simulink library "Compressor_Alpha"  (R2019b)
settings: Solver=ode45  StartTime=0.0  StopTime=10.0  RelTol=1e-3  EnableMultiTasking=on
undefined symbols (not defined in the file): Comp
libraries: $bdroot x4, simulink x1
settings Model: Creator=mbrauer  LastModifiedBy=bhisma
settings DataIOCC: LimitDataPoints=on  SaveFormat=Array  SignalLoggingSaveFormat=ModelDataLogs  ReturnWorkspaceOutputs=off
settings OptimizationCC: LifeSpan=inf
settings DebuggingCC: SolverPrmCheckMsg=warning  MultiTaskDSMMsg=warning  MultiTaskCondExecSysMsg=none  SFUnexpectedBacktrackingDiag=warning  SFNoUnconditionalDefaultTransitionDiag=warning  SFExecutionAtInitializationDiag=none  ArithmeticOperatorsInVariantConditions=warning
settings HardwareCC: ProdBitPerPointer=32  ProdBitPerSizeT=32  ProdBitPerPtrDiffT=32  ProdLargestAtomicFloat=None  ProdIntDivRoundTo=Undefined  ProdEndianess=Unspecified  ProdWordSize=32  ProdHWDeviceType=32-bit Generic
settings ModelReferenceCC: PropagateSignalLabelsOutOfModel=off
settings SFSimCC: SimUseLocalCustomCode=off  CustomCodeUndefinedFunction=UseInterfaceOnly
settings RTWCC: RTWUseLocalCustomCode=off
settings CodeAppCC: StateflowObjectComments=on
settings GRTTargetCC: TargetLangStandard=C89/C90 (ANSI)  GeneratePreprocessorConditionals=Disable all
settings ConfigComp: CovMetricSettings=dw  CovHtmlReporting=on  CovSaveCumulativeToWorkspaceVar=on  CovSaveSingleToWorkspaceVar=on  CovExternalEMLEnable=off

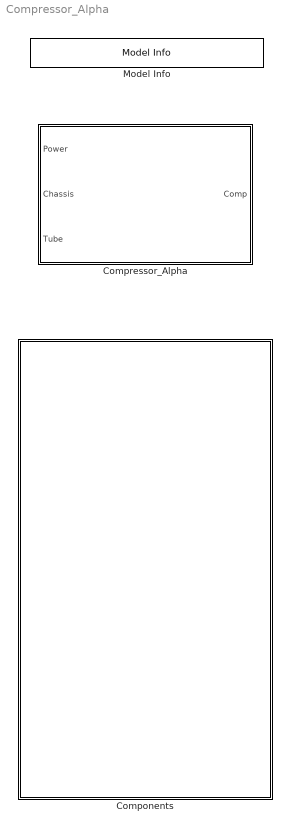
== system Compressor_Alpha ==
  Components : Subsystem
  Compressor_Alpha : Subsystem
  Model Info : simulink/Model-Wide Utilities/Model Info  Frame=on  DisplayStringWithTags=Copyright 2013-2014 The MathWorks, Inc.  HorizontalTextAlignment=Center  LeftAlignmentValue=0.5

== system Compressor_Alpha/Components ==
  Compressor : Subsystem  mask(Compressor){CPR=21, nc=0.75}
      mask prompts: CPR "Compression Ratio"; nc "Efficiency"
      mask help:
      | Basic compressor model, including electric motor.
      |
      | Determines output air pressure and temperature based on defined Compression ratio. Also determines required electrical power.
      mask init:
      | if or(nc > 1,nc<=0)
      |     error('nc should be a value between 0 and 1')
      | end
      | 
      | cp_air = 1e3; 
      | gamma = 1.4;
      mask Display: image('CompressorIcon.png',[80 30 110 140])
  Intercooler : Subsystem  mask(Intercooler){T_air_out=300, eff=0.6}
      mask prompts: T_air_out "Target Output Temperature"; eff "Efficiency"
      mask help:
      | Basic intercooler model, for air to water heat exchange
      |
      | Calculates power to cool input air to desired temperature and converts that heat to water/steam.
      mask init:
      | cp_air      = 1e3;     % kJ/kg/K
      | cp_gas      = 1.996e3; % steam kJ/kg/K
      | cp_liquid   = 4.186e3; % water kJ/kg/K
      | cp_L2G      = 40.7e6/18; % kJ/kg (40.7 kJ/mol / 18 g/mol)
      | T_0         = 273;
      | T_c         = 373;
      | T_max       = 800;
      | maxEnth_liquid = (T_c-T_0)*cp_liquid;
      | minEnth_gas    = maxEnth_liquid+cp_L2G;
      | maxEnth_gas    = minEnth_gas+(T_max-T_c)*cp_gas;
      | if or(eff > 1,eff<=0)
      |     error('eff should be a value between 0 and 1')
      | end
      mask Display: image('Intercooler.png',[60 10 170 180])

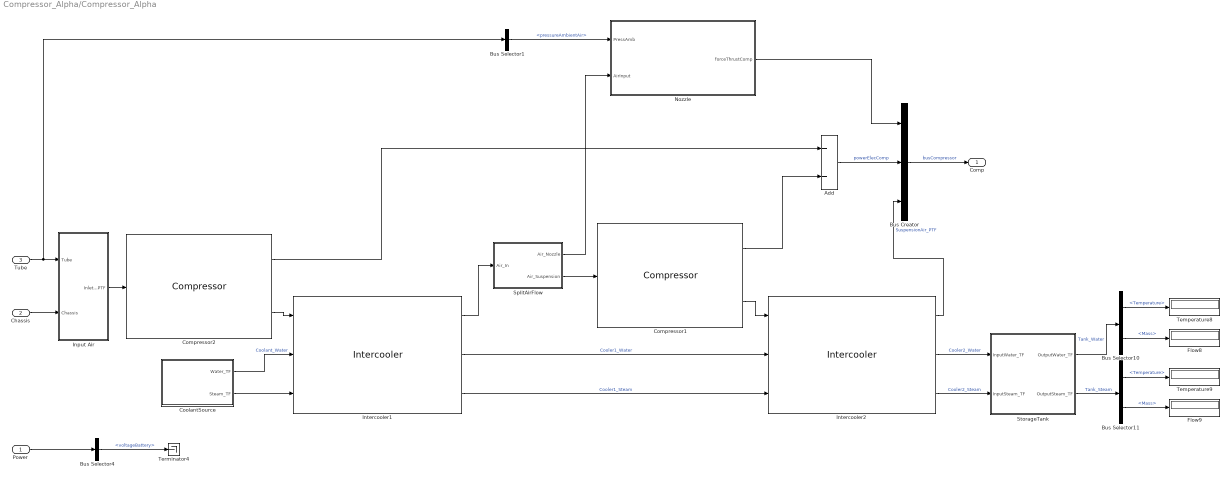
== system Compressor_Alpha/Compressor_Alpha ==
  Power : Inport
  Chassis : Inport  Port=2
  Tube : Inport  Port=3
  Add : Sum  Inputs=--
  Bus Creator : BusCreator  Inputs=3  NonVirtualBus=on
  Bus Selector1 : BusSelector  OutputSignals=pressureAmbientAir
  Bus Selector10 : BusSelector  OutputSignals=Temperature,Mass
  Bus Selector11 : BusSelector  OutputSignals=Temperature,Mass
  Bus Selector4 : BusSelector  OutputSignals=voltageBattery
  Compressor1 : $bdroot/Components/Compressor  CPR=21  nc=0.75
  Compressor2 : $bdroot/Components/Compressor  CPR=21  nc=0.75
  CoolantSource : Subsystem
  Flow8 : Display
      settings: Decimation=100
  Flow9 : Display
      settings: Decimation=100
  Input Air : Subsystem
  Intercooler1 : $bdroot/Components/Intercooler  T_air_out=300  eff=0.6
  Intercooler2 : $bdroot/Components/Intercooler  T_air_out=300  eff=0.6
  Nozzle : Subsystem
  SplitAirFlow : Subsystem
  StorageTank : Subsystem  mask(Liquid/Gas Storage Tank){}
      mask help:
      | This block takes in Flow of a liquid and gas at input temperatures.
      |
      | It accumulates the enthalphy and mass provided and determines a
      | final combination of liquid and gas at proper temperatures.
      |
      | Output should generally be (1) all liquid (2) all gas or (3) a
      | combination of liquid and gas at the boiling point.
      mask init:
      | cp_gas      = 1.996e3; % steam kJ/kg/K
      | cp_liquid   = 4.186e3; % water kJ/kg/K
      | cp_L2G      = 40.7e6/18; % kJ/kg (40.7 kJ/mol / 18 g/mol)
      | T_0         = 273;
      | T_c         = 373;
      | T_max       = 800;
      | maxEnth_liquid = (T_c-T_0)*cp_liquid;
      | minEnth_gas    = maxEnth_liquid+cp_L2G;
      | maxEnth_gas    = minEnth_gas+(T_max-T_c)*cp_gas;
  Temperature8 : Display
      settings: Decimation=100
  Temperature9 : Display
      settings: Decimation=100
  Terminator4 : Terminator
  Comp : Outport
  wires:
  StorageTank/1(OutputWater_TF) -> Bus Selector10/1  "Tank_Water"
  StorageTank/2(OutputSteam_TF) -> Bus Selector11/1  "Tank_Steam"
  Bus Selector11/2 -> Flow9/1  "<Mass>"
  Bus Selector11/1 -> Temperature9/1  "<Temperature>"
  Bus Selector10/2 -> Flow8/1  "<Mass>"
  Bus Selector10/1 -> Temperature8/1  "<Temperature>"
  Intercooler2/3 -> StorageTank/2(InputSteam_TF)  "Cooler2_Steam"
  Intercooler2/2 -> StorageTank/1(InputWater_TF)  "Cooler2_Water"
  Intercooler2/1 -> Bus Creator/3  "SuspensionAir_PTF"
  Compressor1/2 -> Intercooler2/1
  Input Air/1(InletAir_PTF) -> Compressor2/1
  Bus Selector1/1 -> Nozzle/1(PressAmb)  "<pressureAmbientAir>"
  SplitAirFlow/1(Air_Nozzle) -> Nozzle/2(AirInput)
  Intercooler1/1 -> SplitAirFlow/1(Air_In)
  Compressor2/1 -> Add/1
  Compressor1/1 -> Add/2
  Intercooler1/3 -> Intercooler2/3  "Cooler1_Steam"
  SplitAirFlow/2(Air_Suspension) -> Compressor1/1
  Compressor2/2 -> Intercooler1/1
  Bus Selector4/1 -> Terminator4/1  "<voltageBattery>"
  Power/1 -> Bus Selector4/1
  Add/1 -> Bus Creator/2  "powerElecComp"
  Bus Creator/1 -> Comp/1  "busCompressor"
  Nozzle/1(forceThrustComp) -> Bus Creator/1
  Tube/1 -> Bus Selector1/1, Input Air/1(Tube)
  Chassis/1 -> Input Air/2(Chassis)
  CoolantSource/1(Water_TF) -> Intercooler1/2  "Coolant_Water"
  CoolantSource/2(Steam_TF) -> Intercooler1/3
  Intercooler1/2 -> Intercooler2/2  "Cooler1_Water"

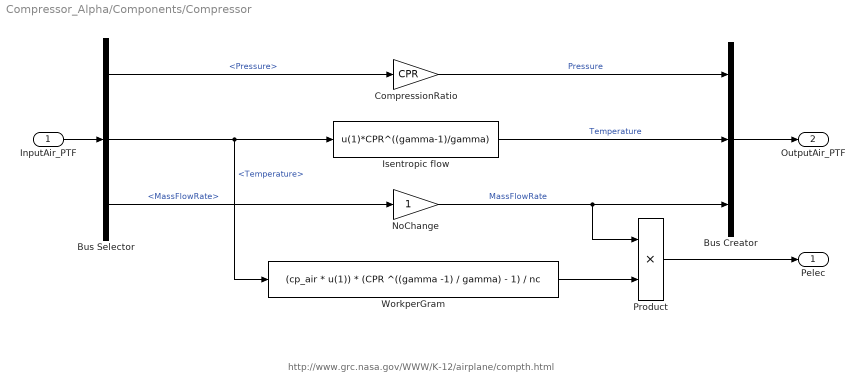
== system Compressor_Alpha/Components/Compressor ==
  note: http://www.grc.nasa.gov/WWW/K-12/airplane/compth.html
  InputAir_PTF : Inport
  Bus Creator : BusCreator  Inputs=3
  Bus Selector : BusSelector  OutputSignals=Pressure,Temperature,MassFlowRate
  CompressionRatio : Gain  Gain=CPR
  Isentropic flow : Fcn  Expr=u(1)*CPR^((gamma-1)/gamma)
  NoChange : Gain
  Product : Product
  WorkperGram : Fcn  Expr=(cp_air * u(1)) * (CPR ^((gamma -1) / gamma) - 1) / nc
  Pelec : Outport
  OutputAir_PTF : Outport  Port=2
  wires:
  Isentropic flow/1 -> Bus Creator/2  "Temperature"
  Bus Selector/2 -> WorkperGram/1, Isentropic flow/1  "<Temperature>"
  Bus Selector/1 -> CompressionRatio/1  "<Pressure>"
  CompressionRatio/1 -> Bus Creator/1  "Pressure"
  WorkperGram/1 -> Product/2
  Product/1 -> Pelec/1
  NoChange/1 -> Product/1, Bus Creator/3  "MassFlowRate"
  Bus Creator/1 -> OutputAir_PTF/1
  InputAir_PTF/1 -> Bus Selector/1
  Bus Selector/3 -> NoChange/1  "<MassFlowRate>"

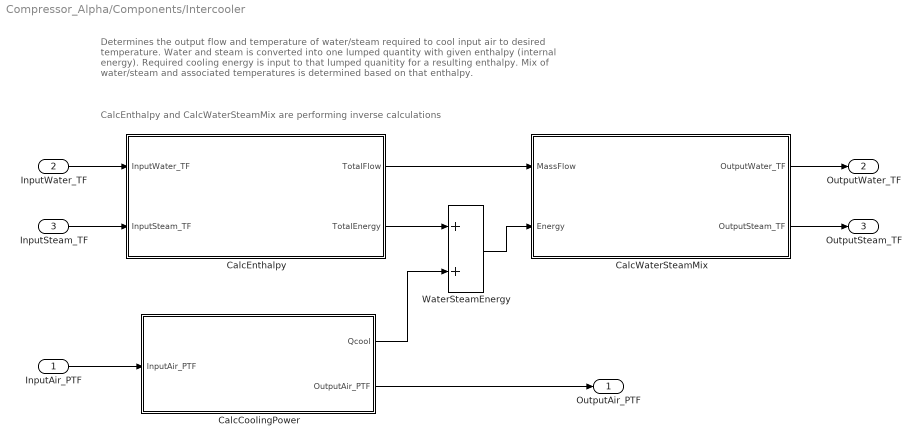
== system Compressor_Alpha/Components/Intercooler ==
  note: CalcEnthalpy and CalcWaterSteamMix are performing inverse calculations
  note: Determines the output flow and temperature of water/steam required to cool input air to desired temperature.
      | Water and steam is converted into one lumped quantity with given enthalpy (internal energy).
      | Required cooling energy is input to that lumped quanitity for a resulting enthalpy.
      | Mix of water/steam and associated temperatures is determined based on that enthalpy.
  InputAir_PTF : Inport
  InputWater_TF : Inport  Port=2
  InputSteam_TF : Inport  Port=3
  CalcCoolingPower : Subsystem
  CalcEnthalpy : Subsystem
  CalcWaterSteamMix : Subsystem
  WaterSteamEnergy : Sum
  OutputAir_PTF : Outport
  OutputWater_TF : Outport  Port=2
  OutputSteam_TF : Outport  Port=3
  wires:
  InputWater_TF/1 -> CalcEnthalpy/1(InputWater_TF)
  InputSteam_TF/1 -> CalcEnthalpy/2(InputSteam_TF)
  InputAir_PTF/1 -> CalcCoolingPower/1(InputAir_PTF)
  CalcCoolingPower/2(OutputAir_PTF) -> OutputAir_PTF/1
  CalcCoolingPower/1(Qcool) -> WaterSteamEnergy/2
  CalcEnthalpy/2(TotalEnergy) -> WaterSteamEnergy/1
  CalcEnthalpy/1(TotalFlow) -> CalcWaterSteamMix/1(MassFlow)
  WaterSteamEnergy/1 -> CalcWaterSteamMix/2(Energy)
  CalcWaterSteamMix/2(OutputSteam_TF) -> OutputSteam_TF/1
  CalcWaterSteamMix/1(OutputWater_TF) -> OutputWater_TF/1

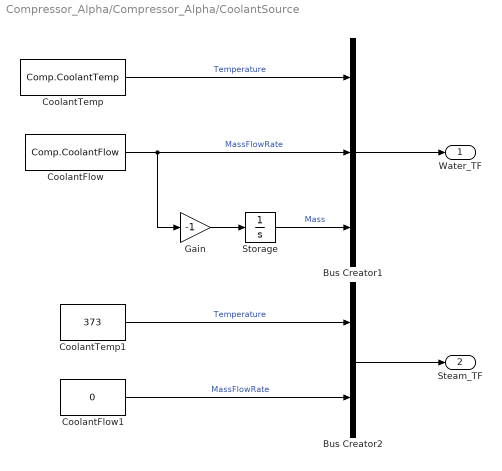
== system Compressor_Alpha/Compressor_Alpha/CoolantSource ==
  Bus Creator1 : BusCreator  Inputs=3
  Bus Creator2 : BusCreator  Inputs=2
  CoolantFlow : Constant  Value=Comp.CoolantFlow
  CoolantFlow1 : Constant  Value=0
  CoolantTemp : Constant  Value=Comp.CoolantTemp
  CoolantTemp1 : Constant  Value=373
  Gain : Gain  Gain=-1
  Storage : Integrator  InitialCondition=Comp.CoolantMass
      settings: AttributesFormatString=IC = %<InitialCondition>
  Water_TF : Outport
  Steam_TF : Outport  Port=2
  wires:
  Gain/1 -> Storage/1
  Storage/1 -> Bus Creator1/3  "Mass"
  CoolantFlow/1 -> Bus Creator1/2, Gain/1  "MassFlowRate"
  CoolantTemp/1 -> Bus Creator1/1  "Temperature"
  Bus Creator1/1 -> Water_TF/1
  Bus Creator2/1 -> Steam_TF/1
  CoolantFlow1/1 -> Bus Creator2/2  "MassFlowRate"
  CoolantTemp1/1 -> Bus Creator2/1  "Temperature"

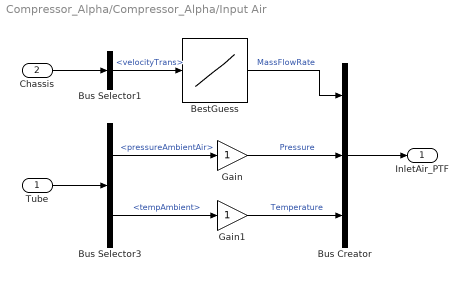
== system Compressor_Alpha/Compressor_Alpha/Input Air ==
  Tube : Inport
  Chassis : Inport  Port=2
  BestGuess : Lookup_n-D  NumberOfTableDimensions=1  BreakpointsForDimension1=[0 100 340 400]  Table=[0.3 0.3 0.49 0.49]  ExtrapMethod=Clip  UseLastTableValue=on  InternalRulePriority=Speed  RndMeth=Simplest  InputSameDT=on
  Bus Creator : BusCreator  Inputs=3
  Bus Selector1 : BusSelector  OutputSignals=velocityTrans
  Bus Selector3 : BusSelector  OutputSignals=pressureAmbientAir,tempAmbient
  Gain : Gain
  Gain1 : Gain
  InletAir_PTF : Outport
  wires:
  Tube/1 -> Bus Selector3/1
  Bus Selector3/1 -> Gain/1  "<pressureAmbientAir>"
  Bus Selector3/2 -> Gain1/1  "<tempAmbient>"
  BestGuess/1 -> Bus Creator/1  "MassFlowRate"
  Chassis/1 -> Bus Selector1/1
  Bus Selector1/1 -> BestGuess/1  "<velocityTrans>"
  Gain/1 -> Bus Creator/2  "Pressure"
  Bus Creator/1 -> InletAir_PTF/1
  Gain1/1 -> Bus Creator/3  "Temperature"

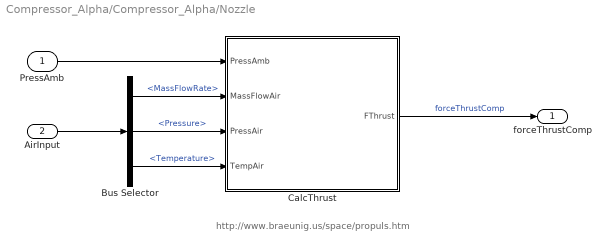
== system Compressor_Alpha/Compressor_Alpha/Nozzle ==
  note: http://www.braeunig.us/space/propuls.htm
  PressAmb : Inport
  AirInput : Inport  Port=2
  Bus Selector : BusSelector  OutputSignals=MassFlowRate,Pressure,Temperature
  CalcThrust : MATLAB Function  TreatAsAtomicUnit=on
  forceThrustComp : Outport
  wires:
  Bus Selector/1 -> CalcThrust/2(MassFlowAir)  "<MassFlowRate>"
  PressAmb/1 -> CalcThrust/1(PressAmb)
  Bus Selector/3 -> CalcThrust/4(TempAir)  "<Temperature>"
  Bus Selector/2 -> CalcThrust/3(PressAir)  "<Pressure>"
  CalcThrust/1(FThrust) -> forceThrustComp/1  "forceThrustComp"
  AirInput/1 -> Bus Selector/1

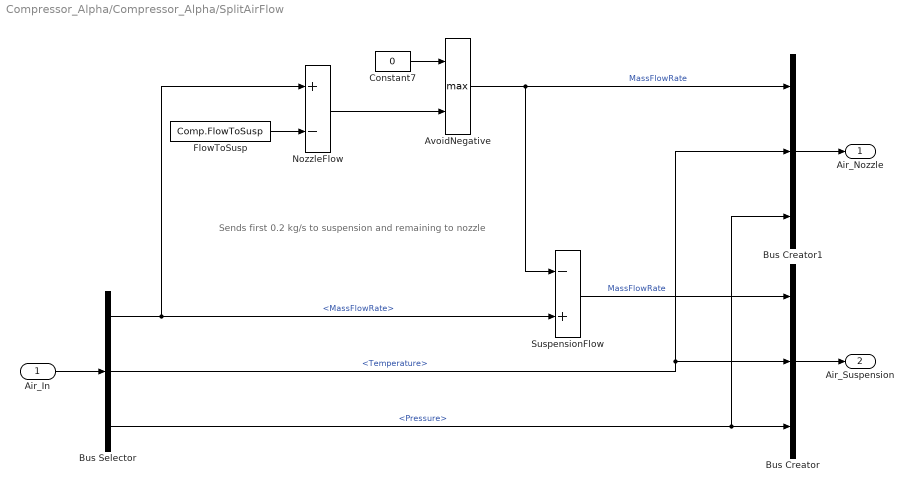
== system Compressor_Alpha/Compressor_Alpha/SplitAirFlow ==
  note: Sends first 0.2 kg/s to suspension and remaining to nozzle
  Air_In : Inport
  AvoidNegative : MinMax  Function=max  Inputs=2
  Bus Creator : BusCreator  Inputs=3
  Bus Creator1 : BusCreator  Inputs=3
  Bus Selector : BusSelector  OutputSignals=MassFlowRate,Temperature,Pressure
  Constant7 : Constant  Value=0
  FlowToSusp : Constant  Value=Comp.FlowToSusp
  NozzleFlow : Sum  Inputs=+-
  SuspensionFlow : Sum  Inputs=-+
  Air_Nozzle : Outport
  Air_Suspension : Outport  Port=2
  wires:
  AvoidNegative/1 -> Bus Creator1/1, SuspensionFlow/1  "MassFlowRate"
  Constant7/1 -> AvoidNegative/1
  NozzleFlow/1 -> AvoidNegative/2
  Bus Selector/1 -> NozzleFlow/1, SuspensionFlow/2  "<MassFlowRate>"
  FlowToSusp/1 -> NozzleFlow/2
  Air_In/1 -> Bus Selector/1
  Bus Creator/1 -> Air_Suspension/1
  Bus Selector/2 -> Bus Creator/2, Bus Creator1/2  "<Temperature>"
  Bus Selector/3 -> Bus Creator1/3, Bus Creator/3  "<Pressure>"
  Bus Creator1/1 -> Air_Nozzle/1
  SuspensionFlow/1 -> Bus Creator/1  "MassFlowRate"

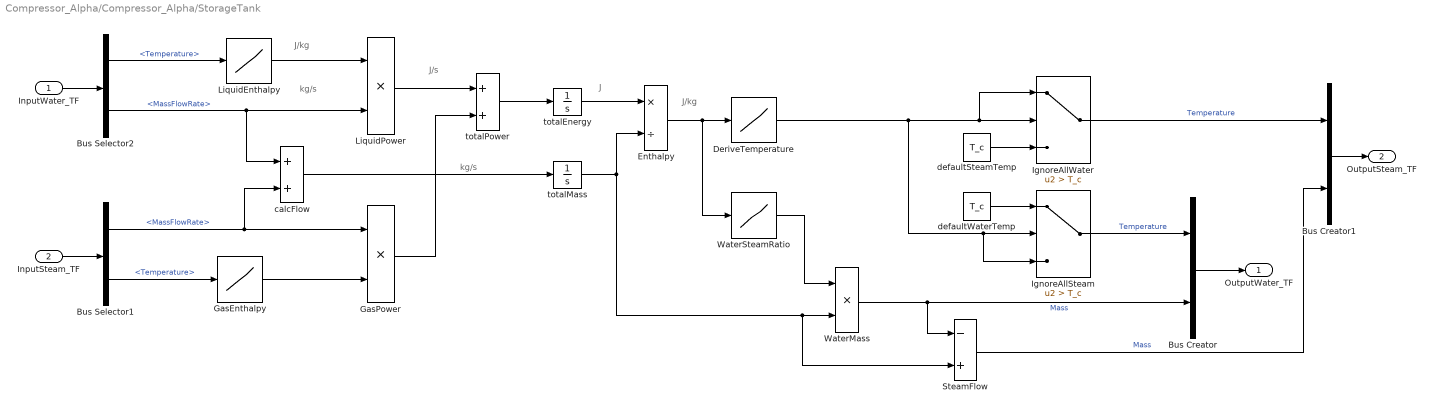
== system Compressor_Alpha/Compressor_Alpha/StorageTank ==
  note: J/kg
  note: kg/s
  note: J/s
  note: J
  note: J/kg
  note: kg/s
  InputWater_TF : Inport
  InputSteam_TF : Inport  Port=2
  Bus Creator : BusCreator  Inputs=2
  Bus Creator1 : BusCreator  Inputs=2
  Bus Selector1 : BusSelector  OutputSignals=MassFlowRate,Temperature
  Bus Selector2 : BusSelector  OutputSignals=Temperature,MassFlowRate
  DeriveTemperature : Lookup_n-D  NumberOfTableDimensions=1  BreakpointsForDimension1=[0 maxEnth_liquid minEnth_gas maxEnth_gas]  Table=[T_0 T_c T_c T_max]  ExtrapMethod=Clip  InternalRulePriority=Speed  RndMeth=Simplest  InputSameDT=on
  Enthalpy : Product  Inputs=*/
  GasEnthalpy : Lookup_n-D  NumberOfTableDimensions=1  BreakpointsForDimension1=[T_c T_max]  Table=[minEnth_gas maxEnth_gas]  ExtrapMethod=Clip  DiagnosticForOutOfRangeInput=Warning  InternalRulePriority=Speed  RndMeth=Simplest  InputSameDT=on
  GasPower : Product  Inputs=**
  IgnoreAllSteam : Switch  Criteria=u2 > Threshold  Threshold=T_c
  IgnoreAllWater : Switch  Criteria=u2 > Threshold  Threshold=T_c
  LiquidEnthalpy : Lookup_n-D  NumberOfTableDimensions=1  BreakpointsForDimension1=[T_0 T_c]  Table=[0 maxEnth_liquid]  ExtrapMethod=Clip  DiagnosticForOutOfRangeInput=Warning  InternalRulePriority=Speed  RndMeth=Simplest  InputSameDT=on
  LiquidPower : Product  Inputs=**
  SteamFlow : Sum  Inputs=-+
  WaterMass : Product
  WaterSteamRatio : Lookup_n-D  NumberOfTableDimensions=1  BreakpointsForDimension1=[0 maxEnth_liquid minEnth_gas maxEnth_gas]  Table=[1 1 0 0]  ExtrapMethod=Clip  UseLastTableValue=on  InternalRulePriority=Speed  RndMeth=Simplest  InputSameDT=on
  calcFlow : Sum
  defaultSteamTemp : Constant  Value=T_c
  defaultWaterTemp : Constant  Value=T_c
  totalEnergy : Integrator
  totalMass : Integrator  InitialCondition=0.01 % avoid div by zero
  totalPower : Sum
  OutputWater_TF : Outport
  OutputSteam_TF : Outport  Port=2
  wires:
  totalEnergy/1 -> Enthalpy/1
  Enthalpy/1 -> DeriveTemperature/1, WaterSteamRatio/1
  DeriveTemperature/1 -> IgnoreAllSteam/3, IgnoreAllSteam/2, IgnoreAllWater/1, IgnoreAllWater/2
  defaultSteamTemp/1 -> IgnoreAllWater/3
  defaultWaterTemp/1 -> IgnoreAllSteam/1
  WaterSteamRatio/1 -> WaterMass/1
  totalMass/1 -> Enthalpy/2, SteamFlow/2, WaterMass/2
  IgnoreAllWater/1 -> Bus Creator1/1  "Temperature"
  IgnoreAllSteam/1 -> Bus Creator/1  "Temperature"
  WaterMass/1 -> SteamFlow/1, Bus Creator/2  "Mass"
  Bus Creator/1 -> OutputWater_TF/1
  Bus Creator1/1 -> OutputSteam_TF/1
  SteamFlow/1 -> Bus Creator1/2  "Mass"
  calcFlow/1 -> totalMass/1
  GasPower/1 -> totalPower/2
  LiquidPower/1 -> totalPower/1
  InputWater_TF/1 -> Bus Selector2/1
  Bus Selector1/2 -> GasEnthalpy/1  "<Temperature>"
  Bus Selector2/1 -> LiquidEnthalpy/1  "<Temperature>"
  Bus Selector2/2 -> calcFlow/1, LiquidPower/2  "<MassFlowRate>"
  InputSteam_TF/1 -> Bus Selector1/1
  GasEnthalpy/1 -> GasPower/2
  LiquidEnthalpy/1 -> LiquidPower/1
  Bus Selector1/1 -> calcFlow/2, GasPower/1  "<MassFlowRate>"
  totalPower/1 -> totalEnergy/1

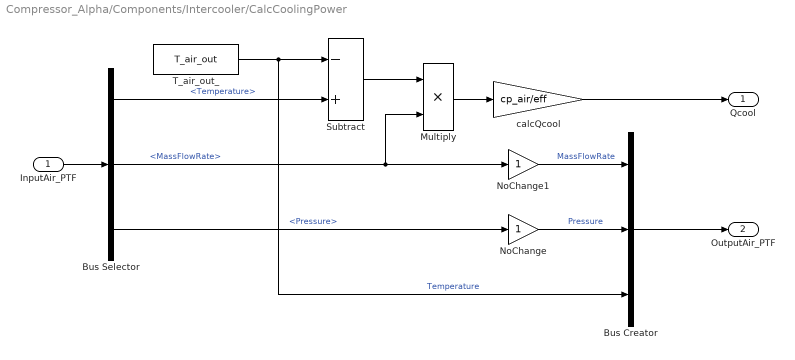
== system Compressor_Alpha/Components/Intercooler/CalcCoolingPower ==
  InputAir_PTF : Inport
  Bus Creator : BusCreator  Inputs=3
  Bus Selector : BusSelector  OutputSignals=Temperature,MassFlowRate,Pressure
  Multiply : Product  Inputs=**
  NoChange : Gain
  NoChange1 : Gain
  Subtract : Sum  Inputs=-+
  T_air_out_ : Constant  Value=T_air_out
  calcQcool : Gain  Gain=cp_air/eff
  Qcool : Outport
  OutputAir_PTF : Outport  Port=2
  wires:
  NoChange1/1 -> Bus Creator/1  "MassFlowRate"
  InputAir_PTF/1 -> Bus Selector/1
  Bus Creator/1 -> OutputAir_PTF/1
  NoChange/1 -> Bus Creator/2  "Pressure"
  Bus Selector/2 -> NoChange1/1, Multiply/2  "<MassFlowRate>"
  Bus Selector/3 -> NoChange/1  "<Pressure>"
  Multiply/1 -> calcQcool/1
  Subtract/1 -> Multiply/1
  calcQcool/1 -> Qcool/1
  Bus Selector/1 -> Subtract/2  "<Temperature>"
  T_air_out_/1 -> Subtract/1, Bus Creator/3  "Temperature"

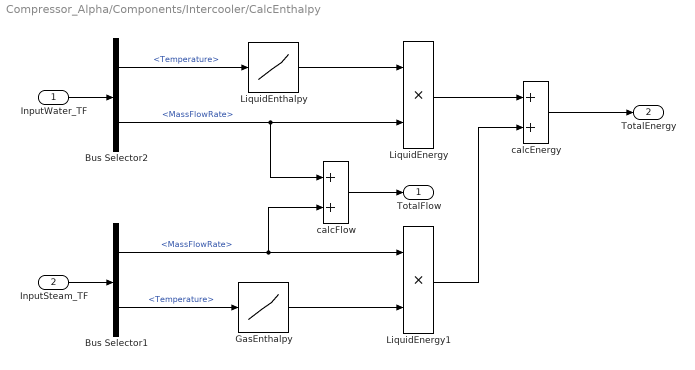
== system Compressor_Alpha/Components/Intercooler/CalcEnthalpy ==
  InputWater_TF : Inport
  InputSteam_TF : Inport  Port=2
  Bus Selector1 : BusSelector  OutputSignals=MassFlowRate,Temperature
  Bus Selector2 : BusSelector  OutputSignals=Temperature,MassFlowRate
  GasEnthalpy : Lookup_n-D  NumberOfTableDimensions=1  BreakpointsForDimension1=[T_c T_max]  Table=[minEnth_gas maxEnth_gas]  ExtrapMethod=Clip  DiagnosticForOutOfRangeInput=Warning  InternalRulePriority=Speed  RndMeth=Simplest  InputSameDT=on
  LiquidEnergy : Product  Inputs=**
  LiquidEnergy1 : Product  Inputs=**
  LiquidEnthalpy : Lookup_n-D  NumberOfTableDimensions=1  BreakpointsForDimension1=[T_0 T_c]  Table=[0 maxEnth_liquid]  ExtrapMethod=Clip  DiagnosticForOutOfRangeInput=Warning  InternalRulePriority=Speed  RndMeth=Simplest  InputSameDT=on
  calcEnergy : Sum
  calcFlow : Sum
  TotalFlow : Outport
  TotalEnergy : Outport  Port=2
  wires:
  calcFlow/1 -> TotalFlow/1
  LiquidEnergy1/1 -> calcEnergy/2
  LiquidEnergy/1 -> calcEnergy/1
  InputWater_TF/1 -> Bus Selector2/1
  Bus Selector1/2 -> GasEnthalpy/1  "<Temperature>"
  Bus Selector2/1 -> LiquidEnthalpy/1  "<Temperature>"
  Bus Selector2/2 -> calcFlow/1, LiquidEnergy/2  "<MassFlowRate>"
  InputSteam_TF/1 -> Bus Selector1/1
  GasEnthalpy/1 -> LiquidEnergy1/2
  LiquidEnthalpy/1 -> LiquidEnergy/1
  Bus Selector1/1 -> calcFlow/2, LiquidEnergy1/1  "<MassFlowRate>"
  calcEnergy/1 -> TotalEnergy/1

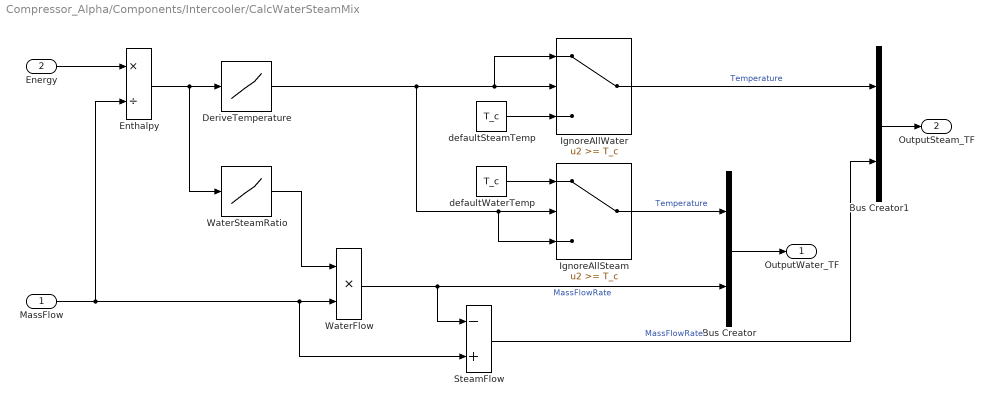
== system Compressor_Alpha/Components/Intercooler/CalcWaterSteamMix ==
  MassFlow : Inport
  Energy : Inport  Port=2
  Bus Creator : BusCreator  Inputs=2
  Bus Creator1 : BusCreator  Inputs=2
  DeriveTemperature : Lookup_n-D  NumberOfTableDimensions=1  BreakpointsForDimension1=[0 maxEnth_liquid minEnth_gas maxEnth_gas]  Table=[T_0 T_c T_c T_max]  ExtrapMethod=Clip  InternalRulePriority=Speed  RndMeth=Simplest  InputSameDT=on
  Enthalpy : Product  Inputs=*/
  IgnoreAllSteam : Switch  Threshold=T_c
  IgnoreAllWater : Switch  Threshold=T_c
  SteamFlow : Sum  Inputs=-+
  WaterFlow : Product
  WaterSteamRatio : Lookup_n-D  NumberOfTableDimensions=1  BreakpointsForDimension1=[0 maxEnth_liquid minEnth_gas maxEnth_gas]  Table=[1 1 0 0]  ExtrapMethod=Clip  UseLastTableValue=on  InternalRulePriority=Speed  RndMeth=Simplest  InputSameDT=on
  defaultSteamTemp : Constant  Value=T_c
  defaultWaterTemp : Constant  Value=T_c
  OutputWater_TF : Outport
  OutputSteam_TF : Outport  Port=2
  wires:
  Energy/1 -> Enthalpy/1
  Enthalpy/1 -> DeriveTemperature/1, WaterSteamRatio/1
  DeriveTemperature/1 -> IgnoreAllSteam/3, IgnoreAllSteam/2, IgnoreAllWater/1, IgnoreAllWater/2
  defaultSteamTemp/1 -> IgnoreAllWater/3
  defaultWaterTemp/1 -> IgnoreAllSteam/1
  WaterSteamRatio/1 -> WaterFlow/1
  MassFlow/1 -> SteamFlow/2, WaterFlow/2, Enthalpy/2
  IgnoreAllWater/1 -> Bus Creator1/1  "Temperature"
  IgnoreAllSteam/1 -> Bus Creator/1  "Temperature"
  WaterFlow/1 -> SteamFlow/1, Bus Creator/2  "MassFlowRate"
  Bus Creator/1 -> OutputWater_TF/1
  Bus Creator1/1 -> OutputSteam_TF/1
  SteamFlow/1 -> Bus Creator1/2  "MassFlowRate"

== matlab function Compressor_Alpha/Nozzle/CalcThrust ==
  data: PressAmb input; MassFlowAir input; PressAir input; TempAir input; FThrust output
function FThrust = fcn(PressAmb, MassFlowAir, PressAir, TempAir  )
%#codegen

% Parameters
gam     = 1.4;  
Rgas    = 287.04;  % J/kg/K

Ve = sqrt(2 * Rgas * gam/(gam-1) * TempAir * (1 - (PressAmb/PressAir)^((gam-1)/gam)));
% Ref http://www.braeunig.us/space/propuls.htm

FThrust = MassFlowAir*Ve;
